simulink model "PID"  (R2024b)
settings: Solver=VariableStepAuto  StartTime=0.0  StopTime=50  RelTol=1e-3
settings Model: Creator=krish  LastModifiedBy=krish

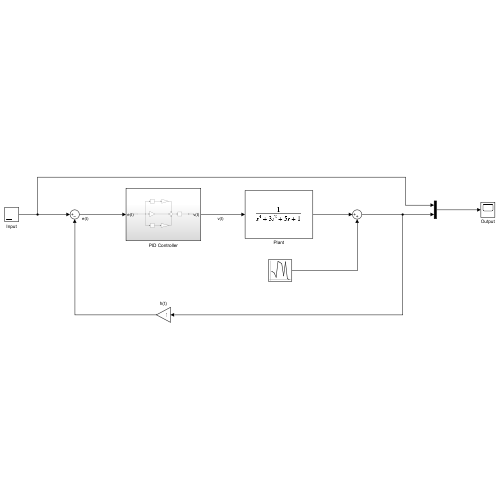
[thumbnail: Simulink's stored preview of the top-level diagram]
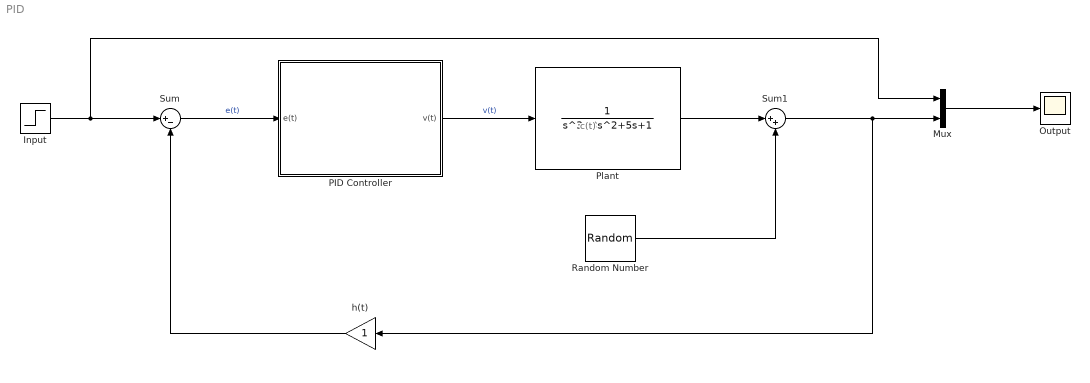
== system PID ==
  note: c(t)
  Input : Step  Time=2  SampleTime=0
  Mux : Mux  Inputs=2
  Output : Scope
  PID Controller : Subsystem
  Plant : TransferFcn  Denominator=[1 3 5 1]
  Random Number : RandomNumber  Variance=0.001  SampleTime=5
  Sum : Sum  Inputs=|+-
  Sum1 : Sum  Inputs=|++
  h(t) : Gain
  wires:
  Input/1 -> Mux/1, Sum/1
  Mux/1 -> Output/1
  h(t)/1 -> Sum/2
  Sum/1 -> PID Controller/1(e(t))  "e(t)"
  PID Controller/1(v(t)) -> Plant/1  "v(t)"
  Plant/1 -> Sum1/1
  Sum1/1 -> h(t)/1, Mux/2
  Random Number/1 -> Sum1/2

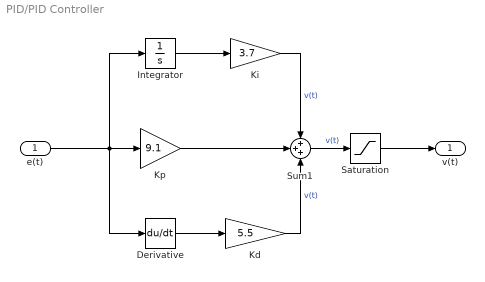
== system PID/PID Controller ==
  e(t) : Inport
  Derivative : Derivative
  Integrator : Integrator
  Kd : Gain  Gain=5.5
  Ki : Gain  Gain=3.7
  Kp : Gain  Gain=9.1
  Saturation : Saturate  UpperLimit=10  LowerLimit=-10
  Sum1 : Sum  Inputs=+++
  v(t) : Outport
  wires:
  Derivative/1 -> Kd/1
  Ki/1 -> Sum1/1  "v(t)"
  Kd/1 -> Sum1/3  "v(t)"
  e(t)/1 -> Derivative/1, Kp/1, Integrator/1
  Saturation/1 -> v(t)/1
  Sum1/1 -> Saturation/1  "v(t)"
  Kp/1 -> Sum1/2
  Integrator/1 -> Ki/1
